simulink model "Robust_2"  (R2024b)
settings: Solver=VariableStepAuto  StartTime=0.0  StopTime=71  RelTol=1e-3
values from neighbouring files (symbols this model uses):
  E_table = E(V_range2,h_funct(Max_Terminal_V_factor),Sharpness_Const)    [Lookup_Tables.m]    (also in Lookup_Tables_and_Initializer.m)
  P_table = 2 * interp1(PWM,POW,1000+u_range*13)    [Lookup_Tables.m]    (also in Lookup_Tables_and_Initializer.m)
  Q_table = interp1(PWM,NTF,1000+u_range*13)    [DuoCopter_EOM2.m]    (also in Lookup_Tables.m; Lookup_Tables_and_Initializer.m)
  T_table = zeros(size(V_range))    [DuoCopter_EOM2.m]    (also in Lookup_Tables.m; Lookup_Tables_and_Initializer.m)
  u_range = 0:1:100    [DuoCopter_EOM2.m]    (also in Lookup_Tables.m; Lookup_Tables_and_Initializer.m)
  V_range = linspace(0,1.25,10)    [DuoCopter_EOM2.m]    (also in Lookup_Tables.m; Lookup_Tables_and_Initializer.m)
  V_range2 = 0:0.01:1.44    [Lookup_Tables.m]    (also in Lookup_Tables_and_Initializer.m)
undefined symbols (not defined in the file or in its folder): DiscIntNeverNeededParam
libraries: simulink x5, slpidlib x3, eeGeneralControl x1, dspstat3 x1, SignalEditorBlockLib x1
settings Model: Creator=sh2323  LastModifiedBy=micha
settings DebuggingCC: AlgebraicLoopMsg=none

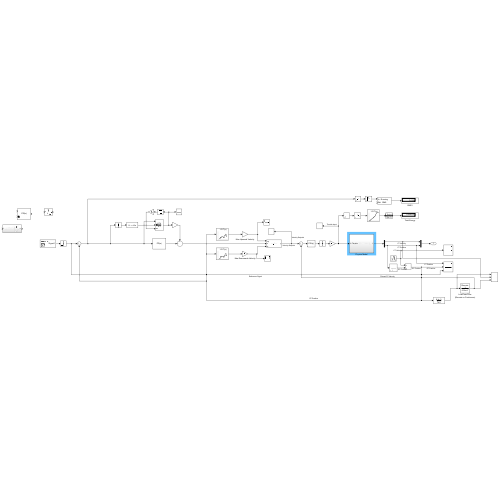
[thumbnail: Simulink's stored preview of the top-level diagram]
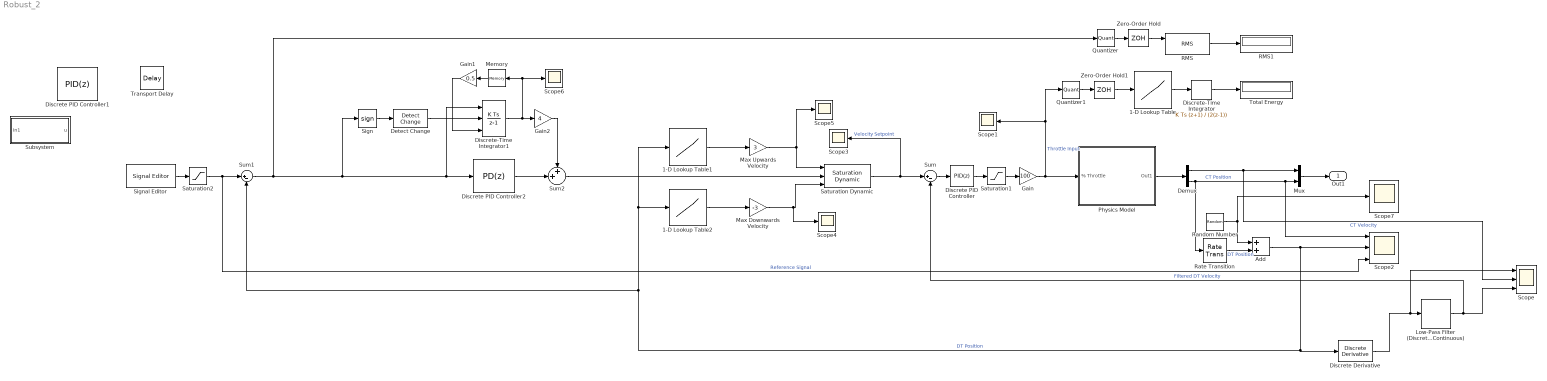
== system Robust_2 ==
  1-D Lookup Table : Lookup_n-D  NumberOfTableDimensions=1  BreakpointsForDimension1=u_range  Table=P_table  InternalRulePriority=Speed  RndMeth=Simplest
  1-D Lookup Table1 : Lookup_n-D  NumberOfTableDimensions=1  BreakpointsForDimension1=V_range2  Table=flip(E_table)  InterpMethod=Nearest  InternalRulePriority=Speed  RndMeth=Simplest
  1-D Lookup Table2 : Lookup_n-D  NumberOfTableDimensions=1  BreakpointsForDimension1=V_range2  Table=E_table  InterpMethod=Nearest  InternalRulePriority=Speed  RndMeth=Simplest
  Add : Sum
  Demux : Demux  Outputs=2
  Detect Change : simulink/Logic and Bit Operations/Detect Change  vinit=0  OutDataTypeStr=boolean
  Discrete Derivative : simulink/Discrete/Discrete Derivative  gainval=1  ICPrevScaledInput=0.0  OutMin=[]  OutMax=[]  OutDataTypeStr=double  OutputDataTypeScalingMode=double  OutDataType=fixdt(1, 16)  OutScaling=2^-10  RndMeth=Simplest  DoSatur=off
  Discrete PID Controller : slpidlib/PID Controller  Controller=PID  Form=Parallel  TimeDomain=Discrete-time  UseExternalTs=off  SampleTime=-1  IntegratorMethod=Forward Euler  FilterMethod=Forward Euler  ControllerParametersSource=internal  P=0.5  I=0.2  UseKiTs=off  D=0  UseExternalDerivativeSource=off  N=100  UseFilter=on  TunerSelectOption=Transfer Function Based (PID Tuner App)  InitialConditionSource=internal  InitialConditionForIntegrator=0  InitialConditionForFilter=0  DifferentiatorICPrevScaledInput=0  ExternalReset=none  TrackingMode=off  Kt=1  LimitOutput=off  SatLimitsSource=internal  UpperSaturationLimit=1  LowerSaturationLimit=0  LinearizeAsGain=off  AntiWindupMode=none  Kb=1  LimitIntegrator=off  UpperIntegratorSaturationLimit=inf  LowerIntegratorSaturationLimit=-inf  POutMin=[]  POutMax=[]  IOutMin=[]  IOutMax=[]  DOutMin=[]  DOutMax=[]  NOutMin=[]  NOutMax=[]  SumOutMin=[]  SumOutMax=[]  SaturationOutMin=[]  SaturationOutMax=[]  PParamMin=[]  PParamMax=[]  IParamMin=[]  IParamMax=[]  DParamMin=[]  DParamMax=[]  NParamMin=[]  NParamMax=[]  KbParamMin=[]  KbParamMax=[]  KtParamMin=[]  KtParamMax=[]  KbOutMin=[]  KbOutMax=[]  KtOutMin=[]  KtOutMax=[]  IntegratorOutMin=[]  IntegratorOutMax=[]  FilterOutMin=[]  FilterOutMax=[]  SumI1OutMin=[]  SumI1OutMax=[]  SumI2OutMin=[]  SumI2OutMax=[]  SumI3OutMin=[]  SumI3OutMax=[]  SumI4OutMin=[]  SumI4OutMax=[]  SumDOutMin=[]  SumDOutMax=[]  DifferentiatorOutMin=[]  DifferentiatorOutMax=[]  FilterDiffOutCoefMin=[]  FilterDiffOutCoefMax=[]  ReciprocalOutMin=[]  ReciprocalOutMax=[]  SumDenOutMin=[]  SumDenOutMax=[]  SumNumOutMin=[]  SumNumOutMax=[]  DivideOutMin=[]  DivideOutMax=[]  UdiffTsProdOutMin=[]  UdiffTsProdOutMax=[]  NTsProdOutMin=[]  NTsProdOutMax=[]  UintegralTsProdOutMin=[]  UintegralTsProdOutMax=[]  UngainTsProdOutMin=[]  UngainTsProdOutMax=[]  ClampingZeroOutDataTypeStr=Inherit: Inherit via back propagation  ClampingZeroOutMin=[]  ClampingZeroOutMax=[]  FilterDenConstantOutDataTypeStr=Inherit: Inherit via back propagation  FilterDenConstantOutMin=[]  FilterDenConstantOutMax=[]  PCopyOutDataTypeStr=Inherit: Inherit via back propagation  PCopyOutMin=[]  PCopyOutMax=[]  NCopyOutDataTypeStr=Inherit: Inherit via back propagation  NCopyOutMin=[]  NCopyOutMax=[]  IntegratorContinuousStateAttributes=''  IntegratorStateMustResolveToSignalObject=off  IntegratorRTWStateStorageClass=Auto  FilterContinuousStateAttributes=''  FilterStateMustResolveToSignalObject=off  FilterRTWStateStorageClass=Auto  ParallelPVariant=InternalParameters  IdealPVariant=Disabled  IVariant=InternalParameters  DVariant=InternalParameters  IntegratorVariant=Discrete  SatVariant=Disabled  AWVariant=Passthrough  PCopyVariant=Disabled  TRVariant=Disabled  FdbkBlocksVariant=Forward  IdealPFdbkVariant=Disabled  SatFdbkVariant=Disabled  DerivativeFilterVariant=ForwardEulerFilter  NVariant=InternalParameters  NCopyVariant=Disabled  FilterICVariant=InternalICsFilter  IntegratorICVariant=InternalICs  ExternalResetVariant=Disabled  TRSumVariant=Passthrough  SumFdbkVariant=Disabled  SumVariant=Sum_PID  TsampFilterVariant=InternalTs  TsampNgainVariant=Passthrough  TsampIntegralVariant=Disabled_SignalSpec  ExternalSaturationOutDataTypeStr=Inherit: Same as second input  DerivativeSourceVariant=ErrorSignal  PreIntVariant=InternalPreInt
      settings: LibrarySourceBlock=simulink/Discrete/Discrete PID Controller
  Discrete PID Controller1 : slpidlib/PID Controller  Controller=PID  Form=Parallel  TimeDomain=Discrete-time  UseExternalTs=off  SampleTime=-1  IntegratorMethod=Forward Euler  FilterMethod=Forward Euler  ControllerParametersSource=internal  P=5  I=4  UseKiTs=off  D=0.1  UseExternalDerivativeSource=off  N=10  UseFilter=on  TunerSelectOption=Transfer Function Based (PID Tuner App)  InitialConditionSource=internal  InitialConditionForIntegrator=0  InitialConditionForFilter=0  DifferentiatorICPrevScaledInput=0  ExternalReset=level  TrackingMode=off  Kt=1  LimitOutput=off  SatLimitsSource=internal  UpperSaturationLimit=inf  LowerSaturationLimit=-inf  LinearizeAsGain=off  AntiWindupMode=none  Kb=1000  LimitIntegrator=off  UpperIntegratorSaturationLimit=1  LowerIntegratorSaturationLimit=-1  POutMin=[]  POutMax=[]  IOutMin=[]  IOutMax=[]  DOutMin=[]  DOutMax=[]  NOutMin=[]  NOutMax=[]  SumOutMin=[]  SumOutMax=[]  SaturationOutMin=[]  SaturationOutMax=[]  PParamMin=[]  PParamMax=[]  IParamMin=[]  IParamMax=[]  DParamMin=[]  DParamMax=[]  NParamMin=[]  NParamMax=[]  KbParamMin=[]  KbParamMax=[]  KtParamMin=[]  KtParamMax=[]  KbOutMin=[]  KbOutMax=[]  KtOutMin=[]  KtOutMax=[]  IntegratorOutMin=[]  IntegratorOutMax=[]  FilterOutMin=[]  FilterOutMax=[]  SumI1OutMin=[]  SumI1OutMax=[]  SumI2OutMin=[]  SumI2OutMax=[]  SumI3OutMin=[]  SumI3OutMax=[]  SumI4OutMin=[]  SumI4OutMax=[]  SumDOutMin=[]  SumDOutMax=[]  DifferentiatorOutMin=[]  DifferentiatorOutMax=[]  FilterDiffOutCoefMin=[]  FilterDiffOutCoefMax=[]  ReciprocalOutMin=[]  ReciprocalOutMax=[]  SumDenOutMin=[]  SumDenOutMax=[]  SumNumOutMin=[]  SumNumOutMax=[]  DivideOutMin=[]  DivideOutMax=[]  UdiffTsProdOutMin=[]  UdiffTsProdOutMax=[]  NTsProdOutMin=[]  NTsProdOutMax=[]  UintegralTsProdOutMin=[]  UintegralTsProdOutMax=[]  UngainTsProdOutMin=[]  UngainTsProdOutMax=[]  ClampingZeroOutDataTypeStr=Inherit: Inherit via back propagation  ClampingZeroOutMin=[]  ClampingZeroOutMax=[]  FilterDenConstantOutDataTypeStr=Inherit: Inherit via back propagation  FilterDenConstantOutMin=[]  FilterDenConstantOutMax=[]  PCopyOutDataTypeStr=Inherit: Inherit via back propagation  PCopyOutMin=[]  PCopyOutMax=[]  NCopyOutDataTypeStr=Inherit: Inherit via back propagation  NCopyOutMin=[]  NCopyOutMax=[]  IntegratorContinuousStateAttributes=''  IntegratorStateMustResolveToSignalObject=off  IntegratorRTWStateStorageClass=Auto  FilterContinuousStateAttributes=''  FilterStateMustResolveToSignalObject=off  FilterRTWStateStorageClass=Auto  ParallelPVariant=InternalParameters  IdealPVariant=Disabled  IVariant=InternalParameters  DVariant=InternalParameters  IntegratorVariant=Discrete  SatVariant=Disabled  AWVariant=Passthrough  PCopyVariant=Disabled  TRVariant=Disabled  FdbkBlocksVariant=Forward  IdealPFdbkVariant=Disabled  SatFdbkVariant=Disabled  DerivativeFilterVariant=ForwardEulerFilter  NVariant=InternalParameters  NCopyVariant=Disabled  FilterICVariant=InternalICsFilter  IntegratorICVariant=InternalICs  ExternalResetVariant=ExternalReset  TRSumVariant=Passthrough  SumFdbkVariant=Disabled  SumVariant=Sum_PID  TsampFilterVariant=InternalTs  TsampNgainVariant=Passthrough  TsampIntegralVariant=Disabled_SignalSpec  ExternalSaturationOutDataTypeStr=Inherit: Same as second input  DerivativeSourceVariant=ErrorSignal  PreIntVariant=InternalPreInt
      settings: LibrarySourceBlock=simulink/Discrete/Discrete PID Controller
  Discrete PID Controller2 : slpidlib/PID Controller  Controller=PD  Form=Parallel  TimeDomain=Discrete-time  UseExternalTs=off  SampleTime=-1  IntegratorMethod=Forward Euler  FilterMethod=Forward Euler  ControllerParametersSource=internal  P=5  I=4  UseKiTs=off  D=0.1  UseExternalDerivativeSource=off  N=10  UseFilter=on  TunerSelectOption=Transfer Function Based (PID Tuner App)  InitialConditionSource=internal  InitialConditionForIntegrator=0  InitialConditionForFilter=0  DifferentiatorICPrevScaledInput=0  ExternalReset=none  TrackingMode=off  Kt=1  LimitOutput=off  SatLimitsSource=internal  UpperSaturationLimit=inf  LowerSaturationLimit=-inf  LinearizeAsGain=off  AntiWindupMode=back-calculation  Kb=10  LimitIntegrator=off  UpperIntegratorSaturationLimit=inf  LowerIntegratorSaturationLimit=-inf  POutMin=[]  POutMax=[]  IOutMin=[]  IOutMax=[]  DOutMin=[]  DOutMax=[]  NOutMin=[]  NOutMax=[]  SumOutMin=[]  SumOutMax=[]  SaturationOutMin=[]  SaturationOutMax=[]  PParamMin=[]  PParamMax=[]  IParamMin=[]  IParamMax=[]  DParamMin=[]  DParamMax=[]  NParamMin=[]  NParamMax=[]  KbParamMin=[]  KbParamMax=[]  KtParamMin=[]  KtParamMax=[]  KbOutMin=[]  KbOutMax=[]  KtOutMin=[]  KtOutMax=[]  IntegratorOutMin=[]  IntegratorOutMax=[]  FilterOutMin=[]  FilterOutMax=[]  SumI1OutMin=[]  SumI1OutMax=[]  SumI2OutMin=[]  SumI2OutMax=[]  SumI3OutMin=[]  SumI3OutMax=[]  SumI4OutMin=[]  SumI4OutMax=[]  SumDOutMin=[]  SumDOutMax=[]  DifferentiatorOutMin=[]  DifferentiatorOutMax=[]  FilterDiffOutCoefMin=[]  FilterDiffOutCoefMax=[]  ReciprocalOutMin=[]  ReciprocalOutMax=[]  SumDenOutMin=[]  SumDenOutMax=[]  SumNumOutMin=[]  SumNumOutMax=[]  DivideOutMin=[]  DivideOutMax=[]  UdiffTsProdOutMin=[]  UdiffTsProdOutMax=[]  NTsProdOutMin=[]  NTsProdOutMax=[]  UintegralTsProdOutMin=[]  UintegralTsProdOutMax=[]  UngainTsProdOutMin=[]  UngainTsProdOutMax=[]  ClampingZeroOutDataTypeStr=Inherit: Inherit via back propagation  ClampingZeroOutMin=[]  ClampingZeroOutMax=[]  FilterDenConstantOutDataTypeStr=Inherit: Inherit via back propagation  FilterDenConstantOutMin=[]  FilterDenConstantOutMax=[]  PCopyOutDataTypeStr=Inherit: Inherit via back propagation  PCopyOutMin=[]  PCopyOutMax=[]  NCopyOutDataTypeStr=Inherit: Inherit via back propagation  NCopyOutMin=[]  NCopyOutMax=[]  IntegratorContinuousStateAttributes=''  IntegratorStateMustResolveToSignalObject=off  IntegratorRTWStateStorageClass=Auto  FilterContinuousStateAttributes=''  FilterStateMustResolveToSignalObject=off  FilterRTWStateStorageClass=Auto  ParallelPVariant=InternalParameters  IdealPVariant=Disabled  IVariant=Disabled  DVariant=InternalParameters  IntegratorVariant=Disabled  SatVariant=Disabled  AWVariant=Disabled  PCopyVariant=Disabled  TRVariant=Disabled  FdbkBlocksVariant=Forward  IdealPFdbkVariant=Disabled  SatFdbkVariant=Disabled  DerivativeFilterVariant=ForwardEulerFilter  NVariant=InternalParameters  NCopyVariant=Disabled  FilterICVariant=InternalICsFilter  IntegratorICVariant=Disabled  ExternalResetVariant=Disabled  TRSumVariant=Passthrough  SumFdbkVariant=Disabled  SumVariant=Sum_PD  TsampFilterVariant=InternalTs  TsampNgainVariant=Passthrough  TsampIntegralVariant=Disabled_SignalSpec  ExternalSaturationOutDataTypeStr=Inherit: Same as second input  DerivativeSourceVariant=ErrorSignal  PreIntVariant=InternalPreInt
      settings: LibrarySourceBlock=simulink/Discrete/Discrete PID Controller
  Discrete-Time Integrator : DiscreteIntegrator  IntegratorMethod=Integration: Trapezoidal  SampleTime=-1  ICPrevOutput=DiscIntNeverNeededParam  ICPrevScaledInput=DiscIntNeverNeededParam
  Discrete-Time Integrator1 : DiscreteIntegrator  ExternalReset=level  InitialConditionSource=external  SampleTime=-1  ICPrevOutput=DiscIntNeverNeededParam  ICPrevScaledInput=DiscIntNeverNeededParam
  Gain : Gain  Gain=100
  Gain1 : Gain  Gain=0.5
  Gain2 : Gain  Gain=4
  Low-Pass Filter (Discrete or Continuous) : eeGeneralControl/Low-Pass Filter (Discrete or Continuous)  K=1  T=0.01  B=inf  A=-inf  init_option=Inherited from block input  x0=0  Ts=-1
  Max Downwards Velocity : Gain  Gain=-3
  Max Upwards Velocity : Gain  Gain=3
  Memory : Memory
  Mux : Mux  Inputs=2
  Physics Model : Subsystem
  Quantizer : Quantizer  QuantizationInterval=0.05
  Quantizer1 : Quantizer  QuantizationInterval=0.05
  RMS : dspstat3/RMS  run=on  directionMode=Each column  dimension=1  reset_popup=Non-zero sample
  RMS1 : Display
  Random Number : RandomNumber  Variance=0.00001  SampleTime=0.05
  Rate Transition : RateTransition  OutPortSampleTime=0.05
  Saturation Dynamic : simulink/Discontinuities/Saturation Dynamic  OutMin=[]  OutMax=[]  OutDataTypeStr=Inherit: Same as second input  OutDataType=fixdt(1, 16)  OutScaling=2^-10  DoSatur=off
  Saturation1 : Saturate  UpperLimit=0.8  LowerLimit=0
  Saturation2 : Saturate  UpperLimit=1.33  LowerLimit=0
  Scope : Scope  NumInputPorts=3
  Scope{1,3..7} (6 alike) : Scope
  Scope2 : Scope  NumInputPorts=3
  Sign : Signum
  Signal Editor : SignalEditorBlockLib/Signal Editor  FileName=C:\Users\micha\Documents\MATLAB\EP2 - Technical\Robust\Tester\samplemission.mat  ActiveScenario=Scenario  ActiveSignal=Signal 1  IsBus=off  OutputBusObjectStr=Bus: BusObject  SampleTime=0  Interpolate=off  ZeroCross=off  OutputAfterFinalValue=Setting to zero  Unit=inherit  PreserveSignalName=on  ApplySigPropsToAllScenarios=on  ApplySigPropsToAllSignals=off
  Subsystem : Subsystem
  Sum : Sum  Inputs=|+-
  Sum1 : Sum  Inputs=|+-
  Sum2 : Sum  Inputs=++|
  Total Energy : Display
  Transport Delay : TransportDelay  DelayTime=0.05*5
  Zero-Order Hold : ZeroOrderHold  SampleTime=-1
  Zero-Order Hold1 : ZeroOrderHold  SampleTime=-1
  Out1 : Outport
  wires:
  Physics Model/1(Out1) -> Demux/1
  Demux/1 -> Scope/2, Mux/1  "CT Velocity"
  Demux/2 -> Rate Transition/1, Mux/2, Scope2/1  "CT Position"
  Mux/1 -> Out1/1
  Add/1 -> Discrete Derivative/1, 1-D Lookup Table1/1, 1-D Lookup Table2/1, Sum1/2, Scope2/2  "DT Position"
  Sum2/1 -> Saturation Dynamic/2
  Gain/1 -> Quantizer1/1, Scope1/1, Physics Model/1(% Throttle)  "Throttle Input"
  Discrete Derivative/1 -> Scope/1, Low-Pass Filter (Discrete or Continuous)/1
  Low-Pass Filter (Discrete or Continuous)/1 -> Scope/3, Sum/2  "Filtered DT Velocity"
  Discrete PID Controller/1 -> Saturation1/1
  Signal Editor/1 -> Saturation2/1
  Saturation1/1 -> Gain/1
  Saturation2/1 -> Scope2/3, Sum1/1  "Reference Signal"
  Discrete-Time Integrator/1 -> Total Energy/1
  RMS/1 -> RMS1/1
  Zero-Order Hold/1 -> RMS/1
  Quantizer1/1 -> Zero-Order Hold1/1
  Quantizer/1 -> Zero-Order Hold/1
  Zero-Order Hold1/1 -> 1-D Lookup Table/1
  Sum/1 -> Discrete PID Controller/1
  1-D Lookup Table/1 -> Discrete-Time Integrator/1
  Saturation Dynamic/1 -> Scope3/1, Sum/1  "Velocity Setpoint"
  Max Upwards Velocity/1 -> Saturation Dynamic/1, Scope5/1
  Max Downwards Velocity/1 -> Scope4/1, Saturation Dynamic/3
  1-D Lookup Table2/1 -> Max Downwards Velocity/1
  1-D Lookup Table1/1 -> Max Upwards Velocity/1
  Sign/1 -> Detect Change/1
  Gain2/1 -> Sum2/1
  Discrete PID Controller2/1 -> Sum2/2
  Discrete-Time Integrator1/1 -> Memory/1, Scope6/1, Gain2/1
  Detect Change/1 -> Discrete-Time Integrator1/2
  Sum1/1 -> Quantizer/1, Sign/1, Discrete-Time Integrator1/1, Discrete PID Controller2/1
  Gain1/1 -> Discrete-Time Integrator1/3
  Memory/1 -> Gain1/1
  Random Number/1 -> Scope7/1, Add/1
  Rate Transition/1 -> Add/2  "DT Position"

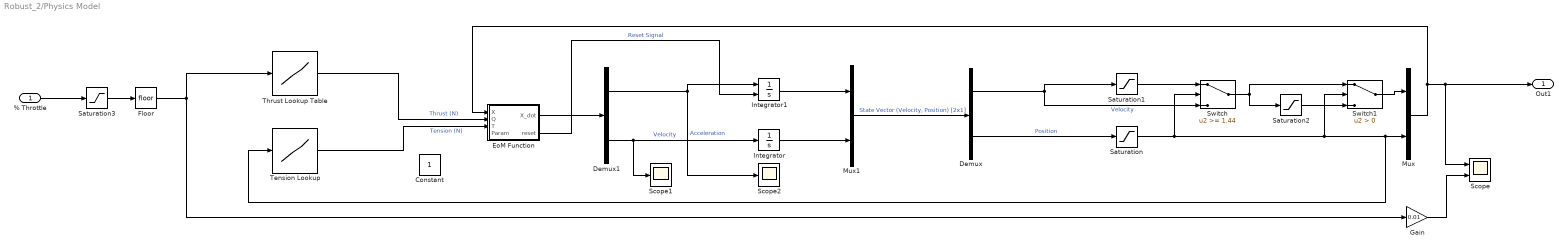
== system Robust_2/Physics Model ==
  % Throttle : Inport
  Constant : Constant
  Demux : Demux  Outputs=2
  Demux1 : Demux  Outputs=2
  EoM Function : MATLAB Function  TreatAsAtomicUnit=on
  Floor : Rounding
  Gain : Gain  Gain=0.01
  Integrator : Integrator
  Integrator1 : Integrator  ExternalReset=rising
  Mux : Mux  Inputs=2
  Mux1 : Mux  Inputs=2
  Saturation : Saturate  UpperLimit=1.44  LowerLimit=0
  Saturation1 : Saturate  UpperLimit=0  LowerLimit=-inf
  Saturation2 : Saturate  UpperLimit=inf  LowerLimit=0
  Saturation3 : Saturate  UpperLimit=100  LowerLimit=0
  Scope : Scope  NumInputPorts=2
  Scope1 : Scope
  Scope2 : Scope
  Switch : Switch  Threshold=1.44  SaturateOnIntegerOverflow=off  InputSameDT=off
  Switch1 : Switch  Criteria=u2 > Threshold  SaturateOnIntegerOverflow=off  InputSameDT=off
  Tension Lookup : Lookup_n-D  NumberOfTableDimensions=1  BreakpointsForDimension1=V_range  Table=T_table  InternalRulePriority=Speed  RndMeth=Simplest
  Thrust Lookup Table : Lookup_n-D  NumberOfTableDimensions=1  BreakpointsForDimension1=u_range  Table=Q_table  InternalRulePriority=Speed  RndMeth=Simplest
  Out1 : Outport
  wires:
  % Throttle/1 -> Saturation3/1
  Mux1/1 -> Demux/1  "State Vector (Velocity, Position) [2x1]"
  Tension Lookup/1 -> EoM Function/3(T)  "Tension (N)"
  Thrust Lookup Table/1 -> EoM Function/2(Q)  "Thrust (N)"
  Demux/2 -> Saturation/1  "Position"
  Mux/1 -> EoM Function/1(X), Scope/1, Out1/1
  Saturation/1 -> Tension Lookup/1, Mux/2, Switch1/2, Switch/2
  Demux/1 -> Switch/3, Saturation1/1  "Velocity"
  Saturation1/1 -> Switch/1
  Switch1/1 -> Mux/1
  Switch/1 -> Saturation2/1, Switch1/1
  Saturation2/1 -> Switch1/3
  EoM Function/1(X_dot) -> Demux1/1
  Demux1/2 -> Integrator/1, Scope1/1  "Velocity"
  Demux1/1 -> Integrator1/1, Scope2/1  "Acceleration"
  Gain/1 -> Scope/2
  Integrator/1 -> Mux1/2
  Integrator1/1 -> Mux1/1
  EoM Function/2(reset) -> Integrator1/2  "Reset Signal"
  Saturation3/1 -> Floor/1
  Floor/1 -> Thrust Lookup Table/1, Gain/1
  ? -> EoM Function/4(Param)

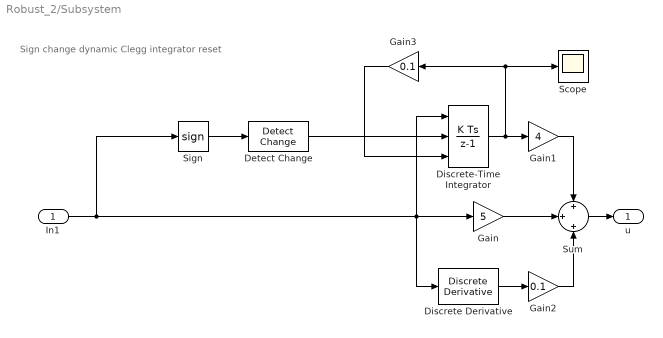
== system Robust_2/Subsystem ==
  note: Sign change dynamic Clegg integrator reset
  In1 : Inport
  Detect Change : simulink/Logic and Bit Operations/Detect Change  vinit=0  OutDataTypeStr=boolean
  Discrete Derivative : simulink/Discrete/Discrete Derivative  gainval=1.0  ICPrevScaledInput=0.0  OutMin=[]  OutMax=[]  OutDataType=fixdt(1, 16)  OutScaling=2^-10  DoSatur=off
  Discrete-Time Integrator : DiscreteIntegrator  ExternalReset=level  InitialConditionSource=external  SampleTime=-1  ICPrevOutput=DiscIntNeverNeededParam  ICPrevScaledInput=DiscIntNeverNeededParam
  Gain : Gain  Gain=5
  Gain1 : Gain  Gain=4
  Gain2 : Gain  Gain=0.1
  Gain3 : Gain  Gain=0.1
  Scope : Scope
  Sign : Signum
  Sum : Sum  Inputs=+|+|+
  u : Outport
  wires:
  Sum/1 -> u/1
  Gain/1 -> Sum/2
  Discrete-Time Integrator/1 -> Scope/1, Gain3/1, Gain1/1
  Gain1/1 -> Sum/1
  Discrete Derivative/1 -> Gain2/1
  Gain2/1 -> Sum/3
  Sign/1 -> Detect Change/1
  In1/1 -> Sign/1, Discrete Derivative/1, Gain/1, Discrete-Time Integrator/1
  Detect Change/1 -> Discrete-Time Integrator/2
  Gain3/1 -> Discrete-Time Integrator/3

== matlab function Robust_2/Physics Model/EoM Function ==
  data: X input; Q input; T input; Param input; X_dot output; reset output
function [X_dot,reset] = fcn(X,Q,T,Param)

%% Robustness parmameters
mu = Param(1);
ST_gram = Param(2);

%% System Parameters

% Constants
g = 9.81;

% Motor choice
m_prop = 0.006;
m_motor = 0.076;
m_esc = 0.042;
m_des = 0.200;
m_cw = 0.050;

% Rail Constraints
x_bottom = 0;
x_top = 1.33;

% Total cart mass (cart mass + arm + propellers + motors + ESC)
m_c = 0.15 + m_des + m_prop + m_motor + m_esc;

% Inertial Mass (cart+counterwieght)
m_i = m_c + m_cw;

% Length dimensions
l_T = 0.035;
l_g = 0.085;
l_c = 0.055;
h = 0.2104;

%% Key Functions

% Friction Force Function  (N)
F = @(Q,T) (2*Q*l_g - g*m_c*l_c - 2*T*l_T )*(mu/h) ;
% Non-Fricative Forces (N)
N = @(Q,T) 2*Q - 2*T - (m_c-m_cw)*g ;
% Static Friction Force (N)
ST = ST_gram / 1000 * 9.81;

%% Equations of Motion

% X(1) ---> Velocity
% X(2) ---> Position

% X_dot(1) ---> Acceleration
% X_dot(2) ---> Velocity

X_dot = zeros(2,1);

% static tolerance

tol = 0.001;
edge_tol = 0.001;

% acceleration at either bound must only be in a specific direction
    % if velocity is greater than 0+tol. , friction acts downwards
    % if velocity is less than 0-tol. friction acts upwards
    % if velocity is within the 'static' range:
        % if non-fricative forces are greater than static force, accel nonzero
        % if non-fricative forces are less than static, accel is zero




if  (X(1) >= -tol) && (X(1) <= tol)

     if abs(N(Q,T)) < ST
        % If non-fricative force can't overcome static friction, no accel
        X_dot(1) = 0;
     elseif N(Q,T) > ST
        % Starting upwards, downwards friction
        X_dot(1) = ( N(Q,T) - ST )/m_i;
     elseif N(Q,T) < -ST
        % Starting upwards, downwards friction
        X_dot(1) = ( N(Q,T) + ST )/m_i;
     end

elseif X(1) > tol
    % Moving Upwards, Downwards Friction
    X_dot(1) = ( N(Q,T) - F(Q,T) )/m_i;

elseif X(1) < -tol
    % Moving Downwards, Upwards Friction
    X_dot(1) = ( N(Q,T) + F(Q,T) )/m_i;
end

reset = 0;

if (X(2) <= x_bottom+edge_tol) && (X_dot(1) < 0)
        X_dot(1) = 0;
elseif (X(2) >= x_top-edge_tol) && (X_dot(1) > 0)
        X_dot(1) = 0; 
end

if (X(2) <= x_bottom+edge_tol) && (X_dot(1) > 0)
        reset = 1;
elseif (X(2) >= x_top-edge_tol) && (X_dot(1) < 0)
        reset = 1; 
end


% Position State Updates
X_dot(2) = X(1);
